simulink model "Realised_inverter_CRD_splittedMCU"  (R2022b)
settings: Solver=ode23tb  StartTime=0.0  StopTime=0.2  MaxStep=2.5e-7  RelTol=1e-3  EnableMultiTasking=on
libraries: spsSeriesRLCBranchLib x18, spsVoltageMeasurementLib x16, spsCurrentMeasurementLib x13, spsMosfetLib x12, spsMeanLib x5, spsIdealSwitchLib x4, spsParallelRLCBranchLib x3, spsDCVoltageSourceLib x2, simulink x2, slpidlib x1, spsThreePhaseSourceLib x1, spspowerguiLib x1
settings Model: SimulationMode=accelerator  Creator=Алексей  LastModifiedBy=alexey
settings SolverCC: ZeroCrossControl=DisableAll  ZeroCrossAlgorithm=Adaptive  AlgebraicLoopSolver=TrustRegion
settings DataIOCC: SaveFormat=Array  SaveOutput=off  SignalLogging=off  DSMLogging=off  SaveTime=off  ReturnWorkspaceOutputs=off
settings OptimizationCC: LifeSpan=inf
settings DebuggingCC: UnderspecifiedInitializationDetection=Classic  MergeDetectMultiDrivingBlocksExec=none  SolverPrmCheckMsg=warning  UnconnectedInputMsg=warning  UnconnectedOutputMsg=warning  UnconnectedLineMsg=warning  AllowSymbolicDim=off  SFUnexpectedBacktrackingDiag=warning  SFNoUnconditionalDefaultTransitionDiag=warning  SFExecutionAtInitializationDiag=none  SFMachineParentedDataDiag=warning  ArithmeticOperatorsInVariantConditions=warning
settings HardwareCC: ProdBitPerPointer=32  ProdBitPerSizeT=32  ProdBitPerPtrDiffT=32  ProdLargestAtomicFloat=None  ProdIntDivRoundTo=Undefined  ProdEndianess=Unspecified  ProdWordSize=32  ProdHWDeviceType=32-bit Generic
settings ModelReferenceCC: EnableRefExpFcnMdlSchedulingChecks=on  PropagateSignalLabelsOutOfModel=off
settings SFSimCC: SimUseLocalCustomCode=off  CustomCodeUndefinedFunction=UseInterfaceOnly
settings RTWCC: RTWUseLocalCustomCode=off  DLArmComputeVersion=19.05
settings CodeAppCC: StateflowObjectComments=on
settings GRTTargetCC: TargetLangStandard=C89/C90 (ANSI)  RTWCAPISignals=on  RTWCAPIParams=on
settings ConfigComp: CovMetricSettings=dw  CovSaveCumulativeToWorkspaceVar=on  CovSaveSingleToWorkspaceVar=on  CovExternalEMLEnable=off  CovSFcnEnable=off
settings SimscapeCC: SimscapeNormalizeSystem=off

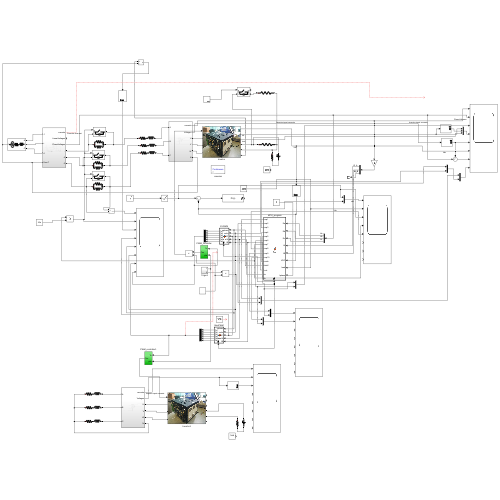
[thumbnail: Simulink's stored preview of the top-level diagram]
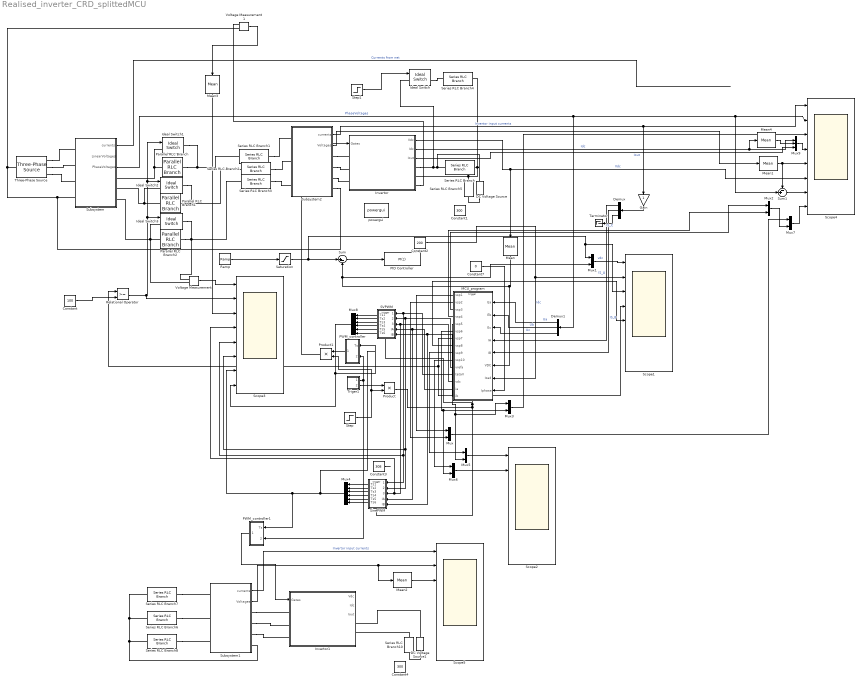
== system Realised_inverter_CRD_splittedMCU ==
  Constant : Constant  Value=100
  Constant1 : Constant  Value=300
  Constant2 : Constant  Value=200
  Constant3 : Constant  Value=308
  Constant4 : Constant  Value=300
  Constant7 : Constant  Value=0
  DC Voltage Source : spsDCVoltageSourceLib/DC Voltage Source  Amplitude=800  Measurements=None
  DC Voltage Source1 : spsDCVoltageSourceLib/DC Voltage Source  Amplitude=800  Measurements=None
  Demux : Demux  Outputs=3
  Demux1 : Demux  Outputs=3
  Gain : Gain
  Ideal Switch : spsIdealSwitchLib/Ideal Switch  Ron=0.001  Lon=0  IC=0  Rs=1e5  Cs=inf  Measurements=on
  Ideal Switch1 : spsIdealSwitchLib/Ideal Switch  Ron=0.001  Lon=0  IC=0  Rs=1e5  Cs=inf  Measurements=off
  Ideal Switch2 : spsIdealSwitchLib/Ideal Switch  Ron=0.001  Lon=0  IC=0  Rs=1e5  Cs=inf  Measurements=off
  Ideal Switch3 : spsIdealSwitchLib/Ideal Switch  Ron=0.001  Lon=0  IC=0  Rs=1e5  Cs=inf  Measurements=off
  Invertor : Subsystem
      mask Display: image('$imagefile'); % Use "Edit Image" on toolstrip to change.
  Invertor1 : Subsystem
      mask Display: image('$imagefile'); % Use "Edit Image" on toolstrip to change.
  MCU_program : MATLAB Function  TreatAsAtomicUnit=on
  Mean : spsMeanLib/Mean  Freq=20000  Vinit=540  Ts=0
  Mean1 : spsMeanLib/Mean  Freq=50000  Vinit=0  Ts=0
  Mean2 : spsMeanLib/Mean  Freq=20000  Vinit=540  Ts=0
  Mean3 : spsMeanLib/Mean  Freq=5000  Vinit=0  Ts=0
  Mean4 : spsMeanLib/Mean  Freq=5000  Vinit=0  Ts=0
  Mux{,1..3,5..7} (7 alike) : Mux  Inputs=2
  Mux4 : Mux  Inputs=6
  Mux8 : Mux  Inputs=6
  Mux9 : Mux  Inputs=3
  PID Controller : slpidlib/PID Controller  Controller=PI  Form=Parallel  TimeDomain=Discrete-time  UseExternalTs=off  SampleTime=10e-6  IntegratorMethod=Forward Euler  FilterMethod=Forward Euler  ControllerParametersSource=internal  P=10  I=1000  UseKiTs=off  D=0  N=100  UseFilter=on  TunerSelectOption=Transfer Function Based (PID Tuner App)  ZeroCross=off  InitialConditionSource=internal  InitialConditionForIntegrator=0  InitialConditionForFilter=0  DifferentiatorICPrevScaledInput=0  ExternalReset=none  TrackingMode=off  Kt=1  LimitOutput=on  SatLimitsSource=internal  UpperSaturationLimit=600  LowerSaturationLimit=0  LinearizeAsGain=on  AntiWindupMode=clamping  Kb=1  LimitIntegrator=off  UpperIntegratorSaturationLimit=inf  LowerIntegratorSaturationLimit=-inf  POutMin=[]  POutMax=[]  IOutMin=[]  IOutMax=[]  DOutMin=[]  DOutMax=[]  NOutMin=[]  NOutMax=[]  SumOutMin=[]  SumOutMax=[]  SaturationOutMin=[]  SaturationOutMax=[]  PParamMin=[]  PParamMax=[]  IParamMin=[]  IParamMax=[]  DParamMin=[]  DParamMax=[]  NParamMin=[]  NParamMax=[]  KbParamMin=[]  KbParamMax=[]  KtParamMin=[]  KtParamMax=[]  KbOutMin=[]  KbOutMax=[]  KtOutMin=[]  KtOutMax=[]  IntegratorOutMin=[]  IntegratorOutMax=[]  FilterOutMin=[]  FilterOutMax=[]  SumI1OutMin=[]  SumI1OutMax=[]  SumI2OutMin=[]  SumI2OutMax=[]  SumI3OutMin=[]  SumI3OutMax=[]  SumI4OutMin=[]  SumI4OutMax=[]  SumDOutMin=[]  SumDOutMax=[]  DifferentiatorOutMin=[]  DifferentiatorOutMax=[]  FilterDiffOutCoefMin=[]  FilterDiffOutCoefMax=[]  ReciprocalOutMin=[]  ReciprocalOutMax=[]  SumDenOutMin=[]  SumDenOutMax=[]  SumNumOutMin=[]  SumNumOutMax=[]  DivideOutMin=[]  DivideOutMax=[]  UdiffTsProdOutMin=[]  UdiffTsProdOutMax=[]  NTsProdOutMin=[]  NTsProdOutMax=[]  UintegralTsProdOutMin=[]  UintegralTsProdOutMax=[]  UngainTsProdOutMin=[]  UngainTsProdOutMax=[]  ClampingZeroOutDataTypeStr=Inherit: Inherit via back propagation  ClampingZeroOutMin=[]  ClampingZeroOutMax=[]  FilterDenConstantOutDataTypeStr=Inherit: Inherit via back propagation  FilterDenConstantOutMin=[]  FilterDenConstantOutMax=[]  PCopyOutDataTypeStr=Inherit: Inherit via back propagation  PCopyOutMin=[]  PCopyOutMax=[]  NCopyOutDataTypeStr=Inherit: Inherit via back propagation  NCopyOutMin=[]  NCopyOutMax=[]  IntegratorContinuousStateAttributes=''  IntegratorStateMustResolveToSignalObject=off  IntegratorRTWStateStorageClass=Auto  FilterContinuousStateAttributes=''  FilterStateMustResolveToSignalObject=off  FilterRTWStateStorageClass=Auto  ParallelPVariant=InternalParameters  IdealPVariant=Disabled  IVariant=InternalParameters  DVariant=Disabled  IntegratorVariant=Discrete  SatVariant=Enabled  AWVariant=DiscClampingParallel  PCopyVariant=Disabled  TRVariant=Disabled  FdbkBlocksVariant=Forward  IdealPFdbkVariant=Disabled  SatFdbkVariant=Disabled  DerivativeFilterVariant=Disabled  NVariant=Disabled  NCopyVariant=Disabled_SignalSpec  FilterICVariant=Disabled  IntegratorICVariant=InternalICs  ExternalResetVariant=Disabled  TRSumVariant=Passthrough  SumFdbkVariant=Disabled  SumVariant=Sum_PI  TsampFilterVariant=InternalTs  TsampNgainVariant=Passthrough  TsampIntegralVariant=Passthrough  ExternalSaturationOutDataTypeStr=Inherit: Same as second input
  PWM_controller : Subsystem
  PWM_controller1 : Subsystem
  Parallel RLC Branch : spsParallelRLCBranchLib/Parallel RLC Branch  LConnTagsString=a  RConnTagsString=__new0  BranchType=RL  Resistance=1000  Inductance=200e-6  SetiL0=off  InitialCurrent=0  Capacitance=1e-6  Setx0=off  InitialVoltage=0  Measurements=None
  Parallel RLC Branch1 : spsParallelRLCBranchLib/Parallel RLC Branch  LConnTagsString=a  RConnTagsString=__new0  BranchType=RL  Resistance=1000  Inductance=200e-6  SetiL0=off  InitialCurrent=0  Capacitance=1e-6  Setx0=off  InitialVoltage=0  Measurements=None
  Parallel RLC Branch2 : spsParallelRLCBranchLib/Parallel RLC Branch  LConnTagsString=a  RConnTagsString=__new0  BranchType=RL  Resistance=1000  Inductance=200e-6  SetiL0=off  InitialCurrent=0  Capacitance=1e-6  Setx0=off  InitialVoltage=0  Measurements=None
  Product : Product
  Product1 : Product
  Ramp : simulink/Sources/Ramp  slope=6500  start=0  InitialOutput=600
  Relational Operator : RelationalOperator  OutDataTypeStr=boolean  RndMeth=Simplest  InputSameDT=off
  SVPWM : MATLAB Function  TreatAsAtomicUnit=on
  Saturation : Saturate  UpperLimit=650  LowerLimit=560
  Scope{1..5} (5 alike) : Scope  NumInputPorts=8
  Series RLC Branch : spsSeriesRLCBranchLib/Series RLC Branch  LConnTagsString=__new0  RConnTagsString=__new0  BranchType=R  Resistance=10  Inductance=1e-3  SetiL0=off  InitialCurrent=0  Capacitance=1e-6  Setx0=off  InitialVoltage=0  Measurements=None
  Series RLC Branch1 : spsSeriesRLCBranchLib/Series RLC Branch  LConnTagsString=__new0  RConnTagsString=__new0  BranchType=RL  Resistance=1e-3  Inductance=200e-6  SetiL0=off  InitialCurrent=0  Capacitance=1e-6  Setx0=off  InitialVoltage=0  Measurements=None
  Series RLC Branch10 : spsSeriesRLCBranchLib/Series RLC Branch  LConnTagsString=__new0  RConnTagsString=__new0  BranchType=R  Resistance=1e-3  Inductance=1e-3  SetiL0=off  InitialCurrent=0  Capacitance=1e-6  Setx0=off  InitialVoltage=0  Measurements=None
  Series RLC Branch2 : spsSeriesRLCBranchLib/Series RLC Branch  LConnTagsString=__new0  RConnTagsString=__new0  BranchType=RL  Resistance=1e-3  Inductance=200e-6  SetiL0=off  InitialCurrent=0  Capacitance=1e-6  Setx0=off  InitialVoltage=0  Measurements=None
  Series RLC Branch3 : spsSeriesRLCBranchLib/Series RLC Branch  LConnTagsString=__new0  RConnTagsString=__new0  BranchType=RL  Resistance=1e-3  Inductance=200e-6  SetiL0=off  InitialCurrent=0  Capacitance=1e-6  Setx0=off  InitialVoltage=0  Measurements=None
  Series RLC Branch4 : spsSeriesRLCBranchLib/Series RLC Branch  LConnTagsString=__new0  RConnTagsString=__new0  BranchType=R  Resistance=2.0e6  Inductance=1e-3  SetiL0=off  InitialCurrent=0  Capacitance=1e-6  Setx0=off  InitialVoltage=0  Measurements=None
  Series RLC Branch5 : spsSeriesRLCBranchLib/Series RLC Branch  LConnTagsString=__new0  RConnTagsString=__new0  BranchType=R  Resistance=1e3  Inductance=1e-3  SetiL0=off  InitialCurrent=0  Capacitance=1e-6  Setx0=off  InitialVoltage=0  Measurements=None
  Series RLC Branch6 : spsSeriesRLCBranchLib/Series RLC Branch  LConnTagsString=__new0  RConnTagsString=__new0  BranchType=RL  Resistance=10  Inductance=700e-6  SetiL0=off  InitialCurrent=0  Capacitance=1e-6  Setx0=off  InitialVoltage=0  Measurements=None
  Series RLC Branch7 : spsSeriesRLCBranchLib/Series RLC Branch  LConnTagsString=__new0  RConnTagsString=__new0  BranchType=RL  Resistance=10  Inductance=700e-6  SetiL0=off  InitialCurrent=0  Capacitance=1e-6  Setx0=off  InitialVoltage=0  Measurements=None
  Series RLC Branch8 : spsSeriesRLCBranchLib/Series RLC Branch  LConnTagsString=__new0  RConnTagsString=__new0  BranchType=RL  Resistance=10  Inductance=700e-6  SetiL0=off  InitialCurrent=0  Capacitance=1e-6  Setx0=off  InitialVoltage=0  Measurements=None
  SinePWM : MATLAB Function  TreatAsAtomicUnit=on
  Step : Step  Time=0  SampleTime=0
  Step1 : Step  Time=0.1  Before=1  After=0  SampleTime=0
  Subsystem : Subsystem
  Subsystem1 : Subsystem
  Subsystem2 : Subsystem
  Sum : Sum  Inputs=|+-
  Sum1 : Sum  Inputs=-+|
  Terminator : Terminator
  Three-Phase Source : spsThreePhaseSourceLib/Three-Phase Source  InternalConnection=Yn  VoltagePhases=on  Voltage=200  PhaseAngle=0  Voltage_phases=[220 220 220]  PhaseAngles_phases=[0 -120 +120]  Frequency=50  NonIdealSource=on  SpecifyImpedance=off  Resistance=1e-6  Inductance=30e-9  ShortCircuitLevel=100e6  BaseVoltage=200  XRratio=7  BusType=swing  Pref=10e3  Qref=0  Prefabc=[10e3, 10e3, 10e3]  Qrefabc=[0, 0, 0]  Qmin=-inf  Qmax=inf
  Triger1 : Subsystem
  Voltage Measurement : spsVoltageMeasurementLib/Voltage Measurement  PhasorSimulation=off  OutputType=Complex  PSBequivalent=0
  Voltage Measurement1 : spsVoltageMeasurementLib/Voltage Measurement  PhasorSimulation=off  OutputType=Complex  PSBequivalent=0
  powergui : spspowerguiLib/powergui  Priority=1  SimulationMode=Continuous  SampleTime=50e-6  frequency=60  Iterations=50  frequencyindice=0  Pbase=100e6  ErrMax=1e-4  UnitsV=kV  UnitsW=MW  buscounter=0  FunctionMessages=off  echomessages=off  EnableUseOfTLC=off  CurrentSourceSwitches=on  DisableSnubberDevices=off  DisableRonSwitches=off  DisableVfSwitches=off  DisplayEquations=off  AutomaticDiscreteSolvers=off  SolverType=Tustin  Interpol=off  ExternalGateDelay=off  methode=off  Ts=0  x0status=blocks  SPID=off  SwTol=0  HookPort=off  NonlinearTolerance=1e-4  nMaxIteration=100  ContinueOnMaxIteration=off  RestoreLinks=warning  ResistiveCurrentMeasurement=off  Frange=[0:2:500]  Ylog=off  Xlog=on  ShowGrid=off  save=off  variable=ZData  structure=SD2  ZoomFFT=on  StartTime=0.7  cycles=10  DisplayStyle=4  fundamental=382  FreqAxis=off  MaxFrequency=50000  frequencyindicesteady=1  RmsSteady=1  display=off
  wires:
  Demux/1 -> MCU_program/4(IA)  "IS_A"
  Demux/2 -> MCU_program/5(IB)  "IS_B"
  MCU_program/2(vsp2) -> Mux/2
  MCU_program/1(vsp1) -> Mux/1
  Triger1/1(1) -> PWM_controller/2(pila), PWM_controller1/2(pila)
  Product1/1 -> Invertor/1(Gates)
  Mux8/1 -> PWM_controller/1(Ts), Scope3/8
  Product/1 -> SVPWM/Trigger, MCU_program/Trigger, SinePWM/Trigger
  Invertor/1(Vdc) -> Scope4/6, Mean/1  "Vdc"
  Invertor/2(Idc) -> Mean4/1, Mux9/1  "Idc"
  Demux/3 -> Terminator/1  "IS_C"
  Demux1/1 -> MCU_program/1(Ea)  "Ua"
  Demux1/2 -> MCU_program/2(Eb)  "Ub"
  Demux1/3 -> MCU_program/3(Ec)  "Uc"
  Subsystem2/1(currents) -> Gain/1, Scope4/1  "Invertor input currents"
  Mux/1 -> Mux7/1
  Subsystem/3(PhaseVoltages) -> Demux1/1, Sum1/2, Scope4/2  "PhaseVoltages"
  MCU_program/4(vsp4) -> Mux2/2
  Constant2/1 -> MCU_program/7(Izad), Scope1/2  "Idc"
  Constant7/1 -> MCU_program/8(Iphase)
  Mux2/1 -> Mux7/2
  MCU_program/3(vsp3) -> Mux2/1
  Triger1/2(2) -> Product/1
  Step/1 -> Product1/2, Product/2
  PWM_controller/1(Tss) -> Product1/1
  MCU_program/5(vsp5) -> Mux5/2, Mux3/1
  MCU_program/6(vsp6) -> Mux3/2, Mux6/2
  Mux3/1 -> Scope4/3
  MCU_program/7(vsp7) -> Relational Operator/1, Scope1/4
  Gain/1 -> Demux/1
  Sum/1 -> PID Controller/1
  Ramp/1 -> Saturation/1
  Step1/1 -> Ideal Switch/1
  Saturation/1 -> Scope1/3, Mux1/1, Sum/1
  Mux1/1 -> Scope1/1  "vdc"
  Subsystem/1(currents) -> ?  "Currents from net"
  MCU_program/8(vsp8) -> Scope1/5
  Mean/1 -> Mux1/2, Sum/2, MCU_program/6(VDC)
  Mux5/1 -> Scope2/1
  Mux6/1 -> Scope2/2
  MCU_program/9(vsp9) -> Mux5/1
  MCU_program/10(vsp10) -> Mux6/1
  Subsystem2/2(Voltages) -> Mean1/1
  Mean1/1 -> Sum1/1, Scope4/5
  Mux7/1 -> Scope4/8
  Sum1/1 -> Scope4/7
  Relational Operator/1 -> Scope3/2, Ideal Switch3/1, Ideal Switch2/1, Ideal Switch1/1
  Constant/1 -> Relational Operator/2
  Voltage Measurement/1 -> Scope3/1
  MCU_program/11(vrefa) -> SinePWM/2(vrefa), Scope3/6, SVPWM/2(vrefa)
  MCU_program/12(tetaV) -> SinePWM/1(vphase), Scope3/5, SVPWM/1(vphase)
  MCU_program/13(vdc) -> Scope3/4, SinePWM/3(VDC), SVPWM/3(VDC)
  MCU_program/14(ia) -> SinePWM/4(IA), SVPWM/4(IA)
  MCU_program/15(ib) -> SinePWM/5(IB), SVPWM/5(IB)
  SVPWM/1(Ts1) -> Mux8/1
  SVPWM/2(Ts2) -> Mux8/2
  SVPWM/3(Ts3) -> Mux8/3
  SVPWM/4(Ts4) -> Mux8/4
  SVPWM/5(Ts5) -> Mux8/5
  SVPWM/6(Ts6) -> Mux8/6
  SinePWM/2(Ts2) -> Mux4/2
  SinePWM/1(Ts1) -> Mux4/1
  SinePWM/3(Ts3) -> Mux4/3
  SinePWM/4(Ts4) -> Mux4/4
  SinePWM/5(Ts5) -> Mux4/5
  SinePWM/6(Ts6) -> Mux4/6
  Constant3/1 -> ?
  Mux4/1 -> PWM_controller1/1(Ts), Scope3/7
  PWM_controller1/1(Tss) -> Invertor1/1(Gates)
  Subsystem1/1(currents) -> Scope5/1  "Invertor input currents"
  Subsystem1/2(Voltages) -> Mean2/1, Scope5/2
  Mean2/1 -> Scope5/3
  Voltage Measurement1/1 -> Mean3/1
  Mean3/1 -> Scope3/3
  Mean4/1 -> Mux9/2
  Mux9/1 -> Scope4/4
  Invertor/3(Iout) -> Mux9/3  "Iout"
  connections:
  Invertor/RConn1 -- DC Voltage Source/RConn1 -- Series RLC Branch/LConn1 -- Ideal Switch/LConn1
  Series RLC Branch/RConn1 -- Invertor/RConn2 -- Series RLC Branch5/LConn1 -- Series RLC Branch4/RConn1
  Three-Phase Source/RConn1 -- Subsystem/LConn1
  Series RLC Branch2/RConn1 -- Subsystem2/LConn2
  Three-Phase Source/RConn2 -- Subsystem/LConn2
  Three-Phase Source/RConn3 -- Subsystem/LConn3
  Series RLC Branch3/RConn1 -- Subsystem2/LConn3
  Series RLC Branch1/RConn1 -- Subsystem2/LConn1
  Parallel RLC Branch1/LConn1 -- Ideal Switch2/LConn1 -- Subsystem/RConn2
  Ideal Switch/RConn1 -- Series RLC Branch4/LConn1
  Parallel RLC Branch/LConn1 -- Subsystem/RConn1 -- Ideal Switch1/LConn1
  Parallel RLC Branch2/LConn1 -- Voltage Measurement/LConn2 -- Ideal Switch3/LConn1 -- Subsystem/RConn3
  Subsystem2/RConn1 -- Invertor/LConn1
  Subsystem2/RConn2 -- Invertor/LConn2
  Subsystem2/RConn3 -- Invertor/LConn3
  Three-Phase Source/LConn1 -- Subsystem2/RConn4 -- Subsystem/LConn4 -- Voltage Measurement1/LConn2
  Parallel RLC Branch/RConn1 -- Ideal Switch1/RConn1 -- Series RLC Branch1/LConn1
  Parallel RLC Branch1/RConn1 -- Ideal Switch2/RConn1 -- Series RLC Branch2/LConn1
  Parallel RLC Branch2/RConn1 -- Ideal Switch3/RConn1 -- Voltage Measurement/LConn1 -- Series RLC Branch3/LConn1
  DC Voltage Source/LConn1 -- Series RLC Branch5/RConn1
  DC Voltage Source1/RConn1 -- Invertor1/RConn1
  Series RLC Branch10/LConn1 -- Invertor1/RConn2
  Series RLC Branch6/RConn1 -- Subsystem1/LConn2
  Series RLC Branch8/RConn1 -- Subsystem1/LConn3
  Series RLC Branch7/RConn1 -- Subsystem1/LConn1
  Subsystem1/RConn1 -- Invertor1/LConn1
  Subsystem1/RConn2 -- Invertor1/LConn2
  Subsystem1/RConn3 -- Invertor1/LConn3
  DC Voltage Source1/LConn1 -- Series RLC Branch10/RConn1
  Series RLC Branch7/LConn1 -- Subsystem1/RConn4 -- Series RLC Branch8/LConn1 -- Series RLC Branch6/LConn1
  Invertor/RConn3 -- Voltage Measurement1/LConn1

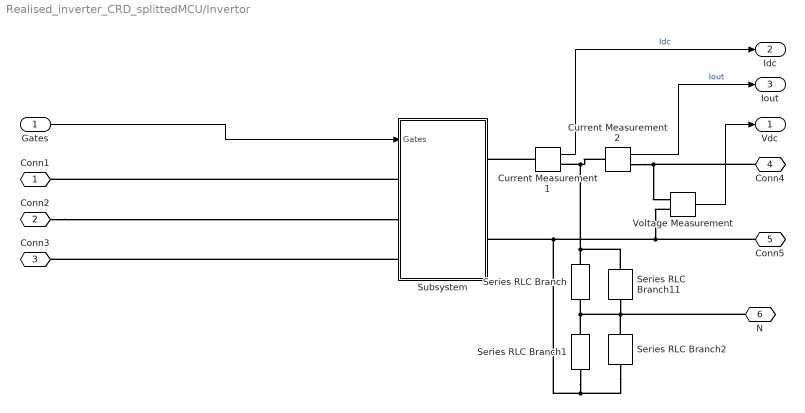
== system Realised_inverter_CRD_splittedMCU/Invertor ==
  Gates : Inport
  Current Measurement1 : spsCurrentMeasurementLib/Current Measurement  PhasorSimulation=off  OutputType=Complex  PSBequivalent=0
  Current Measurement2 : spsCurrentMeasurementLib/Current Measurement  PhasorSimulation=off  OutputType=Complex  PSBequivalent=0
  Series RLC Branch : spsSeriesRLCBranchLib/Series RLC Branch  LConnTagsString=__new0  RConnTagsString=__new0  BranchType=C  Resistance=1  Inductance=1e-3  SetiL0=off  InitialCurrent=0  Capacitance=2500e-6  Setx0=on  InitialVoltage=300  Measurements=None
  Series RLC Branch1 : spsSeriesRLCBranchLib/Series RLC Branch  LConnTagsString=__new0  RConnTagsString=__new0  BranchType=C  Resistance=1  Inductance=1e-3  SetiL0=off  InitialCurrent=0  Capacitance=2500e-6  Setx0=on  InitialVoltage=300  Measurements=None
  Series RLC Branch11 : spsSeriesRLCBranchLib/Series RLC Branch  LConnTagsString=__new0  RConnTagsString=__new0  BranchType=R  Resistance=1e6  Inductance=750e-6  SetiL0=off  InitialCurrent=0  Capacitance=2e-18  Setx0=off  InitialVoltage=0  Measurements=None
  Series RLC Branch2 : spsSeriesRLCBranchLib/Series RLC Branch  LConnTagsString=__new0  RConnTagsString=__new0  BranchType=R  Resistance=1e6  Inductance=750e-6  SetiL0=off  InitialCurrent=0  Capacitance=2e-18  Setx0=off  InitialVoltage=0  Measurements=None
  Subsystem : Subsystem
  Voltage Measurement : spsVoltageMeasurementLib/Voltage Measurement  PhasorSimulation=off  OutputType=Complex  PSBequivalent=0
  Conn1 : PMIOPort  Side=Left
  Conn2 : PMIOPort  Port=2  Side=Left
  Conn3 : PMIOPort  Port=3  Side=Left
  Conn4 : PMIOPort  Port=4  Side=Right
  Conn5 : PMIOPort  Port=5  Side=Right
  N : PMIOPort  Port=6  Side=Right
  Vdc : Outport  VectorParamsAs1DForOutWhenUnconnected=off
  Idc : Outport  Port=2  VectorParamsAs1DForOutWhenUnconnected=off
  Iout : Outport  Port=3  VectorParamsAs1DForOutWhenUnconnected=off
  wires:
  Voltage Measurement/1 -> Vdc/1
  Gates/1 -> Subsystem/1(Gates)
  Current Measurement1/1 -> Idc/1  "Idc"
  Current Measurement2/1 -> Iout/1  "Iout"
  connections:
  Current Measurement1/LConn1 -- Subsystem/RConn1
  Voltage Measurement/LConn2 -- Series RLC Branch2/RConn1 -- Series RLC Branch1/RConn1 -- Subsystem/RConn2 -- Conn5/RConn1
  Subsystem/LConn1 -- Conn1/RConn1
  Conn2/RConn1 -- Subsystem/LConn2
  Subsystem/LConn3 -- Conn3/RConn1
  Conn4/RConn1 -- Current Measurement2/RConn1 -- Voltage Measurement/LConn1
  Current Measurement2/LConn1 -- Series RLC Branch11/LConn1 -- Series RLC Branch/LConn1 -- Current Measurement1/RConn1
  Series RLC Branch1/LConn1 -- N/RConn1 -- Series RLC Branch2/LConn1 -- Series RLC Branch11/RConn1 -- Series RLC Branch/RConn1

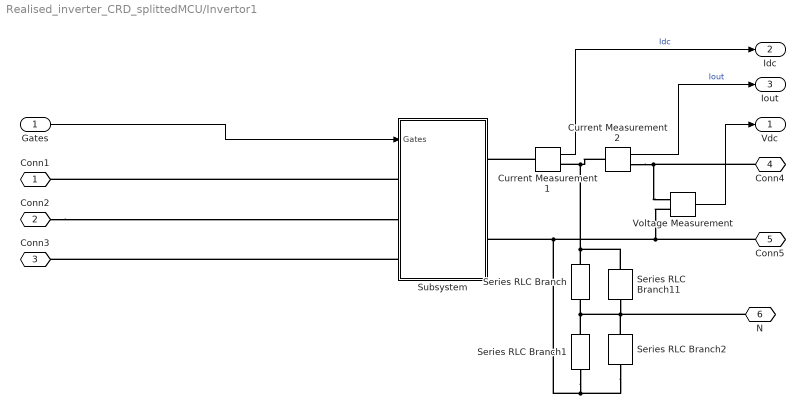
== system Realised_inverter_CRD_splittedMCU/Invertor1 ==
  Gates : Inport
  Current Measurement1 : spsCurrentMeasurementLib/Current Measurement  PhasorSimulation=off  OutputType=Complex  PSBequivalent=0
  Current Measurement2 : spsCurrentMeasurementLib/Current Measurement  PhasorSimulation=off  OutputType=Complex  PSBequivalent=0
  Series RLC Branch : spsSeriesRLCBranchLib/Series RLC Branch  LConnTagsString=__new0  RConnTagsString=__new0  BranchType=C  Resistance=1  Inductance=1e-3  SetiL0=off  InitialCurrent=0  Capacitance=2500e-6  Setx0=on  InitialVoltage=300  Measurements=None
  Series RLC Branch1 : spsSeriesRLCBranchLib/Series RLC Branch  LConnTagsString=__new0  RConnTagsString=__new0  BranchType=C  Resistance=1  Inductance=1e-3  SetiL0=off  InitialCurrent=0  Capacitance=2500e-6  Setx0=on  InitialVoltage=300  Measurements=None
  Series RLC Branch11 : spsSeriesRLCBranchLib/Series RLC Branch  LConnTagsString=__new0  RConnTagsString=__new0  BranchType=R  Resistance=1e6  Inductance=750e-6  SetiL0=off  InitialCurrent=0  Capacitance=2e-18  Setx0=off  InitialVoltage=0  Measurements=None
  Series RLC Branch2 : spsSeriesRLCBranchLib/Series RLC Branch  LConnTagsString=__new0  RConnTagsString=__new0  BranchType=R  Resistance=1e6  Inductance=750e-6  SetiL0=off  InitialCurrent=0  Capacitance=2e-18  Setx0=off  InitialVoltage=0  Measurements=None
  Subsystem : Subsystem
  Voltage Measurement : spsVoltageMeasurementLib/Voltage Measurement  PhasorSimulation=off  OutputType=Complex  PSBequivalent=0
  Conn1 : PMIOPort  Side=Left
  Conn2 : PMIOPort  Port=2  Side=Left
  Conn3 : PMIOPort  Port=3  Side=Left
  Conn4 : PMIOPort  Port=4  Side=Right
  Conn5 : PMIOPort  Port=5  Side=Right
  N : PMIOPort  Port=6  Side=Right
  Vdc : Outport  VectorParamsAs1DForOutWhenUnconnected=off
  Idc : Outport  Port=2  VectorParamsAs1DForOutWhenUnconnected=off
  Iout : Outport  Port=3  VectorParamsAs1DForOutWhenUnconnected=off
  wires:
  Current Measurement2/1 -> Iout/1  "Iout"
  Current Measurement1/1 -> Idc/1  "Idc"
  Gates/1 -> Subsystem/1(Gates)
  Voltage Measurement/1 -> Vdc/1
  connections:
  Series RLC Branch/RConn1 -- Series RLC Branch11/RConn1 -- Series RLC Branch2/LConn1 -- N/RConn1 -- Series RLC Branch1/LConn1
  Current Measurement1/RConn1 -- Series RLC Branch/LConn1 -- Series RLC Branch11/LConn1 -- Current Measurement2/LConn1
  Voltage Measurement/LConn1 -- Current Measurement2/RConn1 -- Conn4/RConn1
  Subsystem/LConn3 -- Conn3/RConn1
  Conn2/RConn1 -- Subsystem/LConn2
  Subsystem/LConn1 -- Conn1/RConn1
  Conn5/RConn1 -- Subsystem/RConn2 -- Series RLC Branch1/RConn1 -- Series RLC Branch2/RConn1 -- Voltage Measurement/LConn2
  Current Measurement1/LConn1 -- Subsystem/RConn1

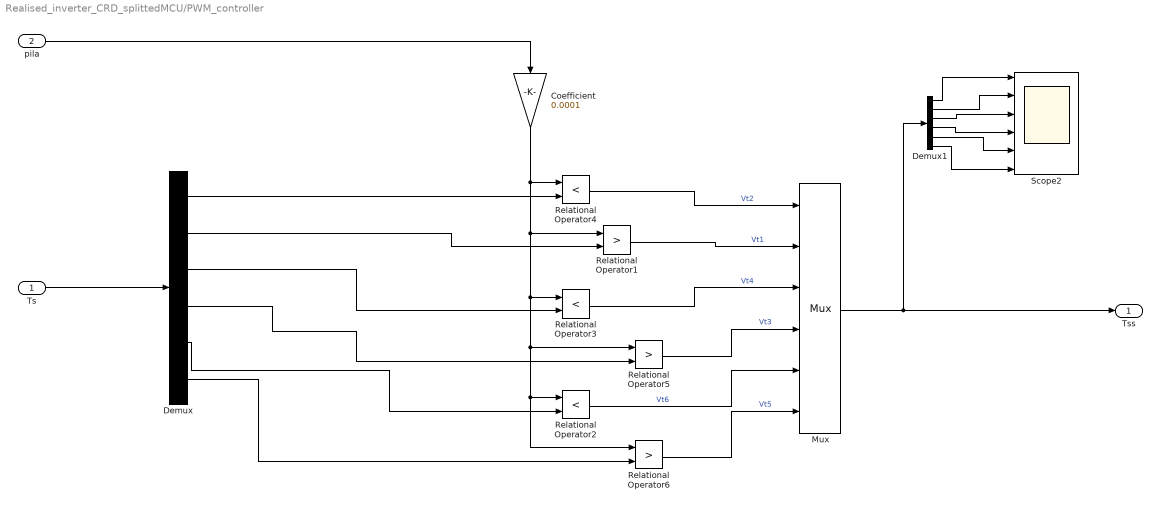
== system Realised_inverter_CRD_splittedMCU/PWM_controller ==
  Ts : Inport
  pila : Inport  Port=2
  Coefficient : Gain  Gain=0.0001
  Demux : Demux  Outputs=6
  Demux1 : Demux  Outputs=6
  Mux : Mux  Inputs=6
  Relational Operator1 : RelationalOperator  Operator=>  OutDataTypeStr=boolean  InputSameDT=off
  Relational Operator2 : RelationalOperator  Operator=<  OutDataTypeStr=boolean  InputSameDT=off
  Relational Operator3 : RelationalOperator  Operator=<  OutDataTypeStr=boolean  InputSameDT=off
  Relational Operator4 : RelationalOperator  Operator=<  OutDataTypeStr=boolean  InputSameDT=off
  Relational Operator5 : RelationalOperator  Operator=>  OutDataTypeStr=boolean  InputSameDT=off
  Relational Operator6 : RelationalOperator  Operator=>  OutDataTypeStr=boolean  InputSameDT=off
  Scope2 : Scope  NumInputPorts=6
  Tss : Outport  VectorParamsAs1DForOutWhenUnconnected=off
  wires:
  Relational Operator4/1 -> Mux/1  "Vt2"
  Demux/3 -> Relational Operator3/2
  Demux/5 -> Relational Operator2/2
  Relational Operator3/1 -> Mux/3  "Vt4"
  Relational Operator2/1 -> Mux/5  "Vt6"
  Ts/1 -> Demux/1
  Coefficient/1 -> Relational Operator1/1, Relational Operator3/1, Relational Operator5/1, Relational Operator2/1, Relational Operator6/1, Relational Operator4/1
  Relational Operator1/1 -> Mux/2  "Vt1"
  Relational Operator5/1 -> Mux/4  "Vt3"
  Relational Operator6/1 -> Mux/6  "Vt5"
  Demux/2 -> Relational Operator1/2
  Demux/4 -> Relational Operator5/2
  Demux/6 -> Relational Operator6/2
  Demux/1 -> Relational Operator4/2
  pila/1 -> Coefficient/1
  Mux/1 -> Tss/1, Demux1/1
  Demux1/2 -> Scope2/2
  Demux1/1 -> Scope2/1
  Demux1/4 -> Scope2/4
  Demux1/5 -> Scope2/5
  Demux1/6 -> Scope2/6
  Demux1/3 -> Scope2/3

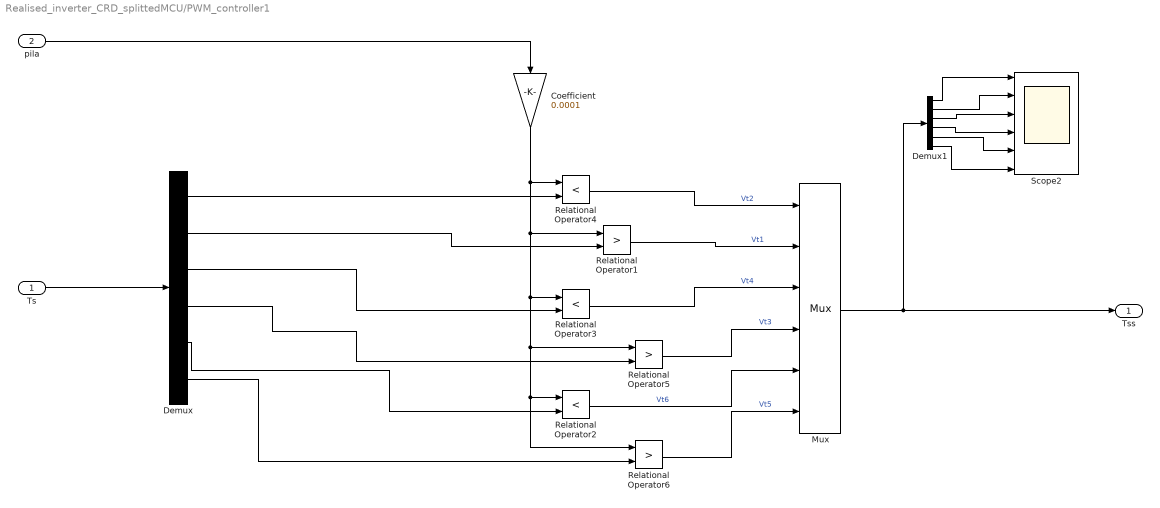
== system Realised_inverter_CRD_splittedMCU/PWM_controller1 ==
  Ts : Inport
  pila : Inport  Port=2
  Coefficient : Gain  Gain=0.0001
  Demux : Demux  Outputs=6
  Demux1 : Demux  Outputs=6
  Mux : Mux  Inputs=6
  Relational Operator1 : RelationalOperator  Operator=>  OutDataTypeStr=boolean  InputSameDT=off
  Relational Operator2 : RelationalOperator  Operator=<  OutDataTypeStr=boolean  InputSameDT=off
  Relational Operator3 : RelationalOperator  Operator=<  OutDataTypeStr=boolean  InputSameDT=off
  Relational Operator4 : RelationalOperator  Operator=<  OutDataTypeStr=boolean  InputSameDT=off
  Relational Operator5 : RelationalOperator  Operator=>  OutDataTypeStr=boolean  InputSameDT=off
  Relational Operator6 : RelationalOperator  Operator=>  OutDataTypeStr=boolean  InputSameDT=off
  Scope2 : Scope  NumInputPorts=6
  Tss : Outport  VectorParamsAs1DForOutWhenUnconnected=off
  wires:
  Demux1/3 -> Scope2/3
  Demux1/6 -> Scope2/6
  Demux1/5 -> Scope2/5
  Demux1/4 -> Scope2/4
  Demux1/1 -> Scope2/1
  Demux1/2 -> Scope2/2
  Mux/1 -> Demux1/1, Tss/1
  pila/1 -> Coefficient/1
  Demux/1 -> Relational Operator4/2
  Demux/6 -> Relational Operator6/2
  Demux/4 -> Relational Operator5/2
  Demux/2 -> Relational Operator1/2
  Relational Operator6/1 -> Mux/6  "Vt5"
  Relational Operator5/1 -> Mux/4  "Vt3"
  Relational Operator1/1 -> Mux/2  "Vt1"
  Coefficient/1 -> Relational Operator4/1, Relational Operator6/1, Relational Operator2/1, Relational Operator5/1, Relational Operator3/1, Relational Operator1/1
  Ts/1 -> Demux/1
  Relational Operator2/1 -> Mux/5  "Vt6"
  Relational Operator3/1 -> Mux/3  "Vt4"
  Demux/5 -> Relational Operator2/2
  Demux/3 -> Relational Operator3/2
  Relational Operator4/1 -> Mux/1  "Vt2"

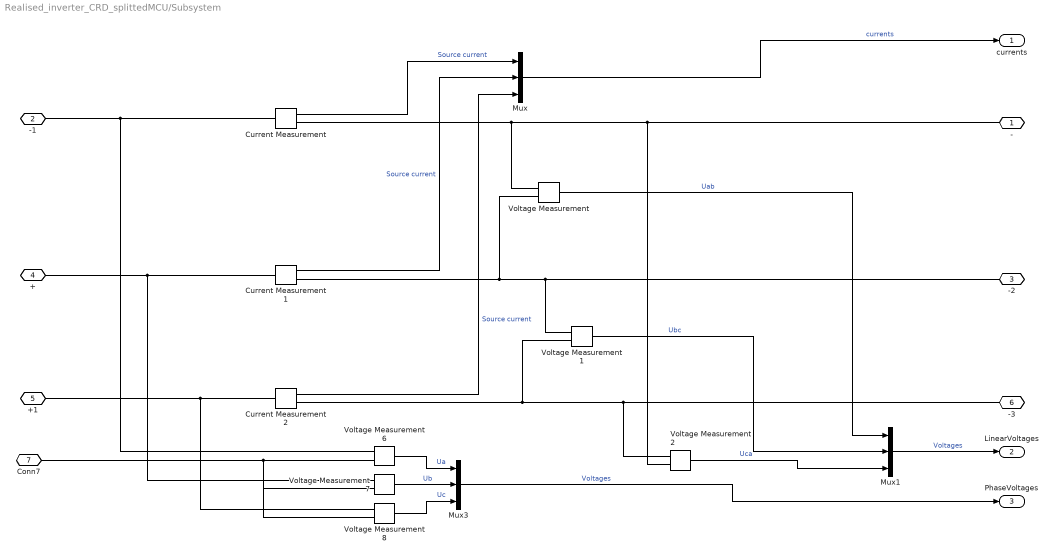
== system Realised_inverter_CRD_splittedMCU/Subsystem ==
  Current Measurement : spsCurrentMeasurementLib/Current Measurement  PhasorSimulation=off  OutputType=Complex  PSBequivalent=0
  Current Measurement1 : spsCurrentMeasurementLib/Current Measurement  PhasorSimulation=off  OutputType=Complex  PSBequivalent=0
  Current Measurement2 : spsCurrentMeasurementLib/Current Measurement  PhasorSimulation=off  OutputType=Complex  PSBequivalent=0
  Mux : Mux  Inputs=3
  Mux1 : Mux  Inputs=3
  Mux3 : Mux  Inputs=3
  Voltage Measurement{,1..2,6..8} (6 alike) : spsVoltageMeasurementLib/Voltage Measurement  PhasorSimulation=off  OutputType=Complex  PSBequivalent=0
  - : PMIOPort  Side=Right
  -1 : PMIOPort  Port=2  Side=Left
  -2 : PMIOPort  Port=3  Side=Right
  + : PMIOPort  Port=4  Side=Left
  +1 : PMIOPort  Port=5  Side=Left
  -3 : PMIOPort  Port=6  Side=Right
  Conn7 : PMIOPort  Port=7  Side=Left
  currents : Outport
  LinearVoltages : Outport  Port=2
  PhaseVoltages : Outport  Port=3
  wires:
  Current Measurement2/1 -> Mux/3  "Source current"
  Current Measurement1/1 -> Mux/2  "Source current"
  Voltage Measurement1/1 -> Mux1/2  "Ubc"
  Voltage Measurement2/1 -> Mux1/3  "Uca"
  Mux/1 -> currents/1  "currents"
  Voltage Measurement/1 -> Mux1/1  "Uab"
  Current Measurement/1 -> Mux/1  "Source current"
  Mux1/1 -> LinearVoltages/1  "Voltages"
  Mux3/1 -> PhaseVoltages/1  "Voltages"
  Voltage Measurement8/1 -> Mux3/3  "Uc"
  Voltage Measurement6/1 -> Mux3/1  "Ua"
  Voltage Measurement7/1 -> Mux3/2  "Ub"
  connections:
  -1/RConn1 -- Voltage Measurement6/LConn1 -- Current Measurement/LConn1
  Current Measurement1/RConn1 -- Voltage Measurement/LConn2 -- -2/RConn1 -- Voltage Measurement1/LConn1
  Current Measurement/RConn1 -- Voltage Measurement/LConn1 -- Voltage Measurement2/LConn2 -- -/RConn1
  Current Measurement2/RConn1 -- Voltage Measurement2/LConn1 -- -3/RConn1 -- Voltage Measurement1/LConn2
  Voltage Measurement6/LConn2 -- Voltage Measurement8/LConn2 -- Voltage Measurement7/LConn2 -- Conn7/RConn1
  +1/RConn1 -- Voltage Measurement8/LConn1 -- Current Measurement2/LConn1
  +/RConn1 -- Voltage Measurement7/LConn1 -- Current Measurement1/LConn1

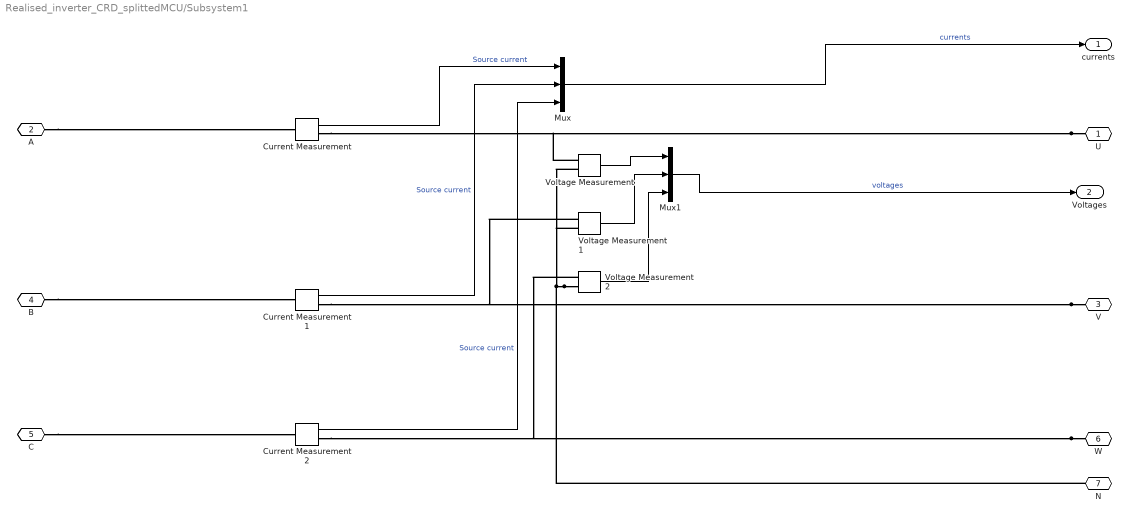
== system Realised_inverter_CRD_splittedMCU/Subsystem1 ==
  Current Measurement : spsCurrentMeasurementLib/Current Measurement  PhasorSimulation=off  OutputType=Complex  PSBequivalent=0
  Current Measurement1 : spsCurrentMeasurementLib/Current Measurement  PhasorSimulation=off  OutputType=Complex  PSBequivalent=0
  Current Measurement2 : spsCurrentMeasurementLib/Current Measurement  PhasorSimulation=off  OutputType=Complex  PSBequivalent=0
  Mux : Mux  Inputs=3
  Mux1 : Mux  Inputs=3
  Voltage Measurement : spsVoltageMeasurementLib/Voltage Measurement  PhasorSimulation=off  OutputType=Complex  PSBequivalent=0
  Voltage Measurement1 : spsVoltageMeasurementLib/Voltage Measurement  PhasorSimulation=off  OutputType=Complex  PSBequivalent=0
  Voltage Measurement2 : spsVoltageMeasurementLib/Voltage Measurement  PhasorSimulation=off  OutputType=Complex  PSBequivalent=0
  U : PMIOPort  Side=Right
  A : PMIOPort  Port=2  Side=Left
  V : PMIOPort  Port=3  Side=Right
  B : PMIOPort  Port=4  Side=Left
  C : PMIOPort  Port=5  Side=Left
  W : PMIOPort  Port=6  Side=Right
  N : PMIOPort  Port=7  Side=Right
  currents : Outport
  Voltages : Outport  Port=2
  wires:
  Voltage Measurement2/1 -> Mux1/3
  Voltage Measurement1/1 -> Mux1/2
  Voltage Measurement/1 -> Mux1/1
  Mux1/1 -> Voltages/1  "voltages"
  Current Measurement2/1 -> Mux/3  "Source current"
  Current Measurement1/1 -> Mux/2  "Source current"
  Mux/1 -> currents/1  "currents"
  Current Measurement/1 -> Mux/1  "Source current"
  connections:
  Voltage Measurement2/LConn2 -- Voltage Measurement1/LConn2 -- Voltage Measurement/LConn2 -- N/RConn1
  A/RConn1 -- Current Measurement/LConn1
  V/RConn1 -- Voltage Measurement1/LConn1 -- Current Measurement1/RConn1
  U/RConn1 -- Voltage Measurement/LConn1 -- Current Measurement/RConn1
  W/RConn1 -- Voltage Measurement2/LConn1 -- Current Measurement2/RConn1
  C/RConn1 -- Current Measurement2/LConn1
  B/RConn1 -- Current Measurement1/LConn1

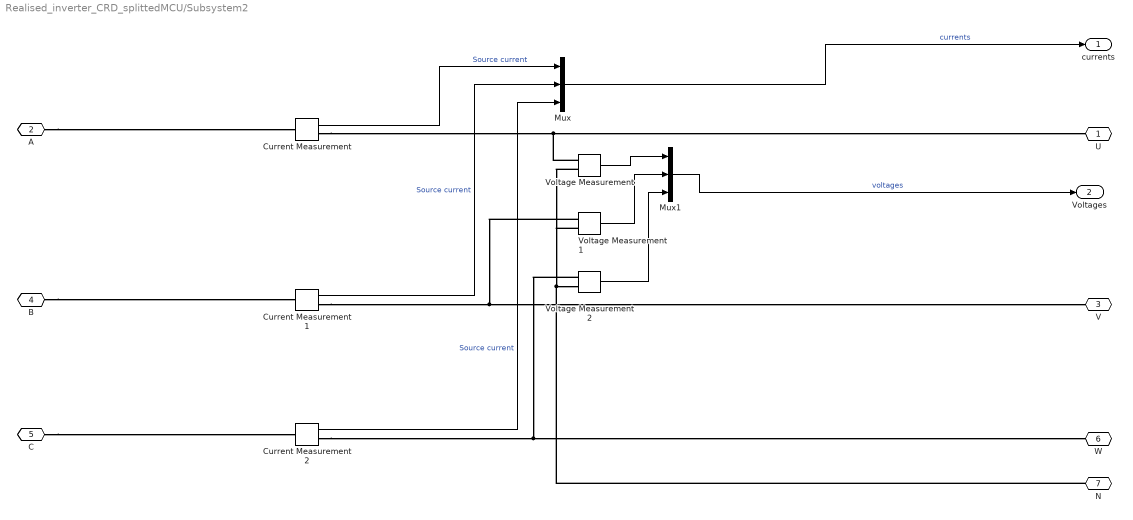
== system Realised_inverter_CRD_splittedMCU/Subsystem2 ==
  Current Measurement : spsCurrentMeasurementLib/Current Measurement  PhasorSimulation=off  OutputType=Complex  PSBequivalent=0
  Current Measurement1 : spsCurrentMeasurementLib/Current Measurement  PhasorSimulation=off  OutputType=Complex  PSBequivalent=0
  Current Measurement2 : spsCurrentMeasurementLib/Current Measurement  PhasorSimulation=off  OutputType=Complex  PSBequivalent=0
  Mux : Mux  Inputs=3
  Mux1 : Mux  Inputs=3
  Voltage Measurement : spsVoltageMeasurementLib/Voltage Measurement  PhasorSimulation=off  OutputType=Complex  PSBequivalent=0
  Voltage Measurement1 : spsVoltageMeasurementLib/Voltage Measurement  PhasorSimulation=off  OutputType=Complex  PSBequivalent=0
  Voltage Measurement2 : spsVoltageMeasurementLib/Voltage Measurement  PhasorSimulation=off  OutputType=Complex  PSBequivalent=0
  U : PMIOPort  Side=Right
  A : PMIOPort  Port=2  Side=Left
  V : PMIOPort  Port=3  Side=Right
  B : PMIOPort  Port=4  Side=Left
  C : PMIOPort  Port=5  Side=Left
  W : PMIOPort  Port=6  Side=Right
  N : PMIOPort  Port=7  Side=Right
  currents : Outport
  Voltages : Outport  Port=2
  wires:
  Current Measurement/1 -> Mux/1  "Source current"
  Mux/1 -> currents/1  "currents"
  Current Measurement1/1 -> Mux/2  "Source current"
  Current Measurement2/1 -> Mux/3  "Source current"
  Mux1/1 -> Voltages/1  "voltages"
  Voltage Measurement/1 -> Mux1/1
  Voltage Measurement1/1 -> Mux1/2
  Voltage Measurement2/1 -> Mux1/3
  connections:
  B/RConn1 -- Current Measurement1/LConn1
  C/RConn1 -- Current Measurement2/LConn1
  Current Measurement2/RConn1 -- Voltage Measurement2/LConn1 -- W/RConn1
  Current Measurement/RConn1 -- Voltage Measurement/LConn1 -- U/RConn1
  Current Measurement1/RConn1 -- Voltage Measurement1/LConn1 -- V/RConn1
  A/RConn1 -- Current Measurement/LConn1
  N/RConn1 -- Voltage Measurement/LConn2 -- Voltage Measurement1/LConn2 -- Voltage Measurement2/LConn2

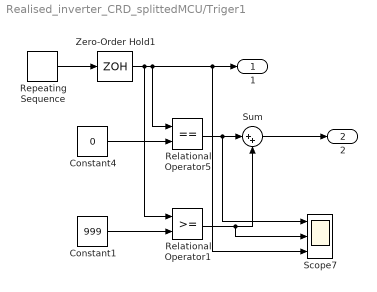
== system Realised_inverter_CRD_splittedMCU/Triger1 ==
  Constant1 : Constant  Value=999
  Constant4 : Constant  Value=0
  Relational Operator1 : RelationalOperator  OutDataTypeStr=boolean  InputSameDT=off
  Relational Operator5 : RelationalOperator  Operator===  OutDataTypeStr=boolean  InputSameDT=off
  Repeating Sequence : simulink/Sources/Repeating Sequence  rep_seq_t=[0 25e-6 50e-6]  rep_seq_y=[0 10000 0]
  Scope7 : Scope  NumInputPorts=3
  Sum : Sum  Inputs=|++
  Zero-Order Hold1 : ZeroOrderHold  SampleTime=2.5e-8
  1 : Outport  VectorParamsAs1DForOutWhenUnconnected=off
  2 : Outport  Port=2  VectorParamsAs1DForOutWhenUnconnected=off
  wires:
  Zero-Order Hold1/1 -> Relational Operator1/1, Relational Operator5/1, Scope7/3, 1/1
  Repeating Sequence/1 -> Zero-Order Hold1/1
  Constant4/1 -> Relational Operator5/2
  Sum/1 -> 2/1
  Constant1/1 -> Relational Operator1/2
  Relational Operator5/1 -> Scope7/1, Sum/1
  Relational Operator1/1 -> Scope7/2, Sum/2

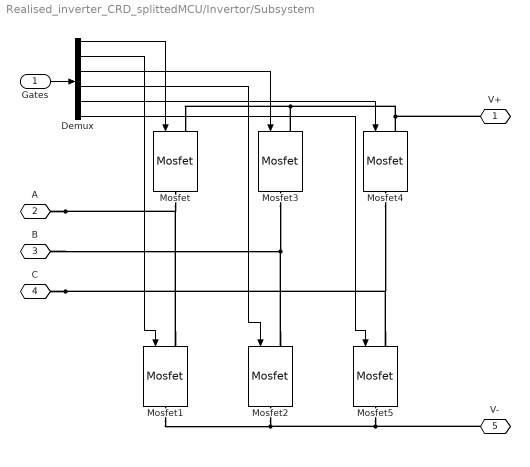
== system Realised_inverter_CRD_splittedMCU/Invertor/Subsystem ==
  Gates : Inport
  Demux : Demux  Outputs=6
  Mosfet : spsMosfetLib/Mosfet  Ron=2e-3  Lon=0  Rd=0.01  Vfd=1e-4  IC=0  Rs=1e5  Cs=inf  Measurements=off
  Mosfet{1..5} (5 alike) : spsMosfetLib/Mosfet  Ron=2e-3  Lon=0  Rd=0.01  Vfd=4  IC=0  Rs=1e5  Cs=inf  Measurements=off
  V+ : PMIOPort  Side=Right
  A : PMIOPort  Port=2  Side=Left
  B : PMIOPort  Port=3  Side=Left
  C : PMIOPort  Port=4  Side=Left
  V- : PMIOPort  Port=5  Side=Right
  wires:
  Demux/4 -> Mosfet2/1
  Demux/2 -> Mosfet1/1
  Demux/5 -> Mosfet4/1
  Demux/3 -> Mosfet3/1
  Demux/6 -> Mosfet5/1
  Demux/1 -> Mosfet/1
  Gates/1 -> Demux/1
  connections:
  C/RConn1 -- Mosfet5/LConn1 -- Mosfet4/RConn1
  V-/RConn1 -- Mosfet5/RConn1 -- Mosfet2/RConn1 -- Mosfet1/RConn1
  B/RConn1 -- Mosfet2/LConn1 -- Mosfet3/RConn1
  V+/RConn1 -- Mosfet3/LConn1 -- Mosfet/LConn1 -- Mosfet4/LConn1
  A/RConn1 -- Mosfet/RConn1 -- Mosfet1/LConn1

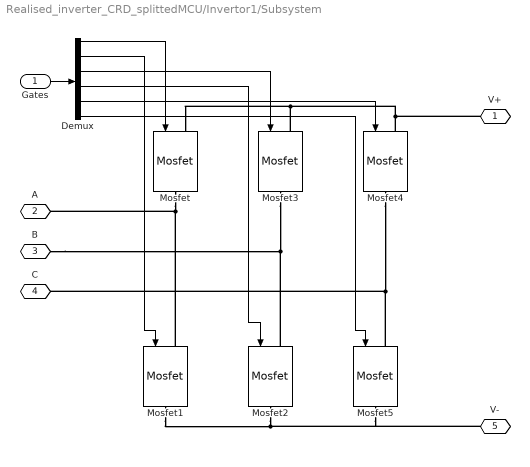
== system Realised_inverter_CRD_splittedMCU/Invertor1/Subsystem ==
  Gates : Inport
  Demux : Demux  Outputs=6
  Mosfet : spsMosfetLib/Mosfet  Ron=2e-3  Lon=0  Rd=0.01  Vfd=1e-4  IC=0  Rs=1e5  Cs=inf  Measurements=off
  Mosfet{1..5} (5 alike) : spsMosfetLib/Mosfet  Ron=2e-3  Lon=0  Rd=0.01  Vfd=4  IC=0  Rs=1e5  Cs=inf  Measurements=off
  V+ : PMIOPort  Side=Right
  A : PMIOPort  Port=2  Side=Left
  B : PMIOPort  Port=3  Side=Left
  C : PMIOPort  Port=4  Side=Left
  V- : PMIOPort  Port=5  Side=Right
  wires:
  Gates/1 -> Demux/1
  Demux/1 -> Mosfet/1
  Demux/6 -> Mosfet5/1
  Demux/3 -> Mosfet3/1
  Demux/5 -> Mosfet4/1
  Demux/2 -> Mosfet1/1
  Demux/4 -> Mosfet2/1
  connections:
  Mosfet1/LConn1 -- Mosfet/RConn1 -- A/RConn1
  Mosfet4/LConn1 -- Mosfet/LConn1 -- Mosfet3/LConn1 -- V+/RConn1
  Mosfet3/RConn1 -- Mosfet2/LConn1 -- B/RConn1
  Mosfet1/RConn1 -- Mosfet2/RConn1 -- Mosfet5/RConn1 -- V-/RConn1
  Mosfet4/RConn1 -- Mosfet5/LConn1 -- C/RConn1

== matlab function Realised_inverter_CRD_splittedMCU/MCU_program ==
  data: Ea input; Eb input; Ec input; IA input; IB input; vsp1 output; vsp2 output; vsp3 output; vsp4 output; VDC input; Izad input; Iphase input; vsp5 output; vsp6 output; vsp7 output; vsp8 output; vsp9 output; vsp10 output; vrefa output; tetaV output; vdc output; ia output; ib output
  events: trigger input RISING_EDGE_EVENT
function [vsp1,vsp2,vsp3,vsp4,vsp5,vsp6,vsp7, vsp8, vsp9, vsp10,vrefa,tetaV, vdc,ia,ib] = fcn(Ea,Eb,Ec,IA,IB,VDC, Izad, Iphase)
%время 1/2 ШИМ период
dt = 10e-6;
R = 1e-3;
L = 270e-6;


kureactp = 7.5;
kureacti = kureactp * R / L;

kuactp = 7.5;
kuacti = kuactp * R / L;


persistent Ureactint;
if isempty(Ureactint)
    Ureactint = 0;
end 
persistent Uactint;
if isempty(Uactint)
    Uactint = 0;
end 


%Преобразования Кларка
Ialfa = -IA;
Ibeta = -(2*IB+IA)/sqrt(3);


Ealfa = Ea;
Ebeta = (Eb - Ec)/sqrt(3);

E_ampl = sqrt(Ealfa^2+Ebeta^2);
teta=acos(Ealfa/E_ampl)*sign(Ebeta)+(sign(Ebeta)-1)*(-pi);

% реальные значения ЭДС сети Eact И Ereact. При этом всегда должно
% получаться, что Ereact = 0
Eact = Ealfa*cos(teta) + Ebeta*sin(teta);
Ereact = Ebeta*cos(teta) - Ealfa*sin(teta); 

%реальные значения токов Iact и Ireact, полученные через  угол и оси альфа,бета 
Iact = Ialfa*cos(teta) + Ibeta*sin(teta);
Iact = -Iact; %Перевод в систему координат инвертора - для него поглащается активный ток сети
Ireact = Ibeta*cos(teta) - Ialfa*sin(teta); 

Ireact_zad = -Izad * sin(Iphase);
%ПИ-регулятор для напряжения по оси react
direact = Ireact_zad - Ireact;
Ureactpr = direact * kureactp;
Ureactint = Ureactint + direact*kureacti*dt;


Iact_zad = Izad * cos(Iphase);
%ПИ-регулятор для напряжения по оси act
diact = Iact_zad - Iact;
Uactpr = diact*kuactp;
Uactint = Uactint + diact * kuacti * dt;

  
U_react  =Ureactpr + Ureactint;                    
U_act = Uactpr + Uactint;

Um = (2/3)*VDC/sqrt(U_react^2+U_act^2)*0.85;

if(Um<1)
  U_react = U_react * Um;
  U_act = U_act * Um;
end


U_react = Ereact + U_react;
U_act = Eact - U_act;


Ua0 = U_act*cos(teta) - U_react*sin(teta);
Ub0 = U_act*sin(teta) + U_react*cos(teta);



vrefa = sqrt(Ua0^2 + Ub0^2);
tetaV = acos(Ua0/vrefa)*sign(Ub0) + (sign(Ub0) - 1)*(-pi);

ia= IA;
ib = IB;
vdc = VDC;

vsp1 = Ealfa;
vsp2 = Ua0;
vsp3 = Ebeta;
vsp4 = Ub0;
vsp5 = U_act;%Iact_zad;
vsp6 = U_react;%Ireact_zad;
vsp7 = Iact;
vsp8 = Ireact;
vsp9 = Eact;
vsp10 = Ereact;


return

== matlab function Realised_inverter_CRD_splittedMCU/SVPWM ==
  data: vphase input; vrefa input; VDC input; IA input; IB input; Ts1 output; Ts2 output; Ts3 output; Ts4 output; Ts5 output; Ts6 output
  events: trigger input RISING_EDGE_EVENT
function [Ts1,Ts2,Ts3,Ts4,Ts5,Ts6] = fcn(vphase,vrefa,VDC,IA,IB)
%время 1/2 ШИМ периода
dt=100e-6;


%алгоритм формирования векторной ШИМ  мертвым веменем dead [мкс]
dead=0.0;
dead=dead/(dt*1e6);
a=vphase;
v2=vrefa*1.5;
if a>=0 && a<pi/3 
    n=1;
elseif  a>=pi/3 && a<2*pi/3 
    n=2;
elseif  a>=2*pi/3 && a<pi 
    n=3;
elseif  a>=pi && a<4*pi/3 
    n=4;
elseif  a>=4*pi/3 && a<5*pi/3 
    n=5;
else n=6;

end

a_cor=a-(n-1)*pi/3;

T1 = (v2/VDC)*sin(pi/3-a_cor)/sin(pi/3);
T2 = (v2/VDC)*sin(a_cor)/sin(pi/3);
T0=1-T1-T2;
Ta1=0; Ta3=0; Ta5=0; 
switch n
    case 1
        
        Ta1=T1+T2+T0/2;
        
        Ta3=T2+T0/2;
       
        Ta5=T0/2;
       
    case 2
        
        Ta1=T1+T0/2;
        
        Ta3=T1+T2+T0/2;
    
        Ta5=T0/2;       
        
    case 3
        
        Ta1=T0/2;
       
        Ta3=T1+T2+T0/2;
       
        Ta5=T2+T0/2;    
        
    case 4
        
        Ta1=T0/2;
       
        Ta3=T1+T0/2;
       
        Ta5=T1+T2+T0/2;   
       
    case 5
        
        Ta1=T2+T0/2;
        
        Ta3=T0/2;
        
        Ta5=T1+T2+T0/2;     
        
    case 6
        
        Ta1=T1+T2+T0/2;
        
        Ta3=T0/2;
     
        Ta5=T1+T0/2;    
        
end;


Ts1=(Ta1)+dead/2; 
Ts3=(Ta3)+dead/2; 
Ts5=(Ta5)+dead/2;
Ts2=(Ta1)-dead/2; 
Ts4=(Ta3)-dead/2; 
Ts6=(Ta5)-dead/2;


if (IA>0) 
    Ts1=Ts1+dead/2;
    Ts2=Ts2+dead/2;
else
    Ts1=Ts1-dead/2;
    Ts2=Ts2-dead/2;           
end;
if (IB>0) 
    Ts3=Ts3+dead/2;
    Ts4=Ts4+dead/2;
else
    Ts3=Ts3-dead/2;
    Ts4=Ts4-dead/2; 
end;  
if ((-IA-IB)>0) 
    Ts5=Ts5+dead/2;
    Ts6=Ts6+dead/2;
else
    Ts5=Ts5-dead/2;
    Ts6=Ts6-dead/2;           
end;


return;

== matlab function Realised_inverter_CRD_splittedMCU/SinePWM ==
  data: vphase input; vrefa input; VDC input; IA input; IB input; Ts1 output; Ts2 output; Ts3 output; Ts4 output; Ts5 output; Ts6 output
  events: trigger input RISING_EDGE_EVENT
function [Ts1,Ts2,Ts3,Ts4,Ts5,Ts6] = fcn(vphase,vrefa,VDC,IA,IB)
%время 1/2 ШИМ периода
dt=100e-6;


%алгоритм формирования векторной ШИМ  мертвым веменем dead [мкс]
dead=0.0;
dead=dead/(dt*1e6);

compensate = 0;



Ta1 = 0.5 + (vrefa/(VDC*1/2))*cos(vphase)/2;
Ta3 = 0.5 + (vrefa/(VDC*1/2))*cos(vphase + 4*pi/3)/2;
Ta5 = 0.5 + (vrefa/(VDC*1/2))*cos(vphase + 2*pi/3)/2;


Ts1=(Ta1)+dead/2; 
Ts3=(Ta3)+dead/2; 
Ts5=(Ta5)+dead/2;
Ts2=(Ta1)-dead/2; 
Ts4=(Ta3)-dead/2; 
Ts6=(Ta5)-dead/2;

if compensate == 1
    if (IA>0) 
        Ts1=Ts1+dead/2;
        Ts2=Ts2+dead/2;
    else
        Ts1=Ts1-dead/2;
        Ts2=Ts2-dead/2;           
    end
    if (IB>0) 
        Ts3=Ts3+dead/2;
        Ts4=Ts4+dead/2;
    else
        Ts3=Ts3-dead/2;
        Ts4=Ts4-dead/2; 
    end
    if ((-IA-IB)>0) 
        Ts5=Ts5+dead/2;
        Ts6=Ts6+dead/2;
    else
        Ts5=Ts5-dead/2;
        Ts6=Ts6-dead/2;           
    end
end


return;
